simulink model "cantxrx"  (R2020b)
settings: Solver=FixedStepDiscrete  StartTime=0.0  StopTime=Inf  FixedStep=1e-3  RelTol=1e-3  EnableMultiTasking=on
model workspace (MAT data in the model file):
  state_control = Simulink.Signal
  state_control.DataType = 'uint8'
  state_control.Dimensions = -1
  state_control.DimensionsMode = 'Fixed'
  state_control.Complexity = 'real'
  state_control.SampleTime = -1
  state_control.SamplingMode = 'auto'
  state_control.InitialValue = '99'
libraries: simulink x12, hdlsllib x10, c280xlib x3, canmsglib x2, c2837xDlib x2, c2000lib x1
settings Model: ExtModeTrigDuration=8  OrderedModelArguments=off  Creator=sgcesuser2  LastModifiedBy=sgcesuser2
settings SolverCC: AutoInsertRateTranBlk=on
settings OptimizationCC: DefaultUnderspecifiedDataType=single  EnhancedBackFolding=on  PassReuseOutputArgsAs=Individual arguments  MaxStackSize=1024  OptimizeBlockOrder=speed  DifferentSizesBufferReuse=on  OptimizationCustomize=off  DenormalBehavior=FlushToZero  EfficientTunableParamExpr=on
settings DebuggingCC: ParameterTunabilityLossMsg=error
settings HardwareCC: ProdBitPerChar=16  ProdBitPerInt=16  ProdBitPerPointer=32  ProdBitPerSizeT=32  ProdBitPerPtrDiffT=32  ProdLargestAtomicInteger=Integer  ProdLargestAtomicFloat=None  ProdWordSize=16  ProdLongLongMode=on  ProdHWDeviceType=Texas Instruments->C2000
settings SFSimCC: MATLABDynamicMemAlloc=off
settings RTWCC: Description=Embedded Coder  SystemTargetFile=ert.tlc  HardwareBoard=TI Delfino F28379D LaunchPad  TemplateMakefile=ert_default_tmf  CustomHeaderCode="#include \"can_defines.h\""  Toolchain=Texas Instruments Code Composer Studio (C2000)
settings CodeAppCC: ForceParamTrailComments=on  IgnoreCustomStorageClasses=off  OperatorAnnotations=on  SimulinkDataObjDesc=on  SFDataObjDesc=on  InsertBlockDesc=on
settings ERTTargetCC: CodeReplacementLibrary=TI C28x  ExtModeTransport=3  ExtModeStaticAllocSize=10000

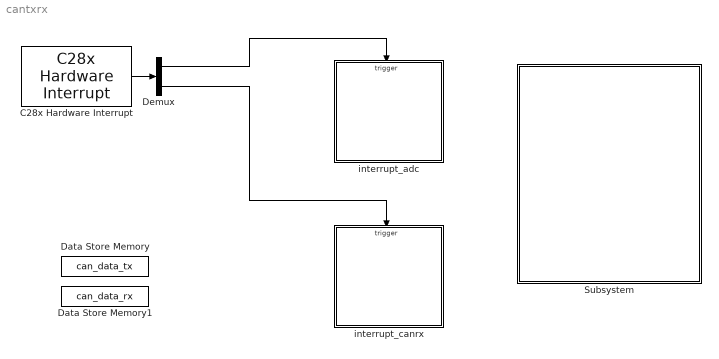
== system cantxrx ==
  C28x Hardware Interrupt : c2000lib/Scheduling/C28x Hardware Interrupt  irqnumbers=[1 9]  pienumbers=[1 7]  irqpriorities=[30 26]  irqpreempts=[0 1]  showinput=off  dspchiptype=C280X
      settings: SourceProductBaseCode=TIC2000
  Data Store Memory : DataStoreMemory  DataStoreName=can_data_tx  ReadBeforeWriteMsg=warning  WriteAfterWriteMsg=warning  WriteAfterReadMsg=warning  ShowAdditionalParam=off  Dimensions=[1 8]
  Data Store Memory1 : DataStoreMemory  DataStoreName=can_data_rx  ReadBeforeWriteMsg=warning  WriteAfterWriteMsg=warning  WriteAfterReadMsg=warning  ShowAdditionalParam=off  Dimensions=[1 8]
  Demux : Demux  Outputs=2
  Subsystem : Subsystem  TreatAsAtomicUnit=on  SystemSampleTime=1
  interrupt_adc : Subsystem  TreatAsAtomicUnit=on
      settings: RTWFcnNameOpts=Use subsystem name  RTWFileNameOpts=Use subsystem name
  interrupt_canrx : Subsystem  TreatAsAtomicUnit=on
      settings: RTWFcnNameOpts=Use subsystem name  RTWFileNameOpts=Use subsystem name
  wires:
  Demux/2 -> interrupt_canrx/Trigger
  Demux/1 -> interrupt_adc/Trigger
  C28x Hardware Interrupt/1 -> Demux/1

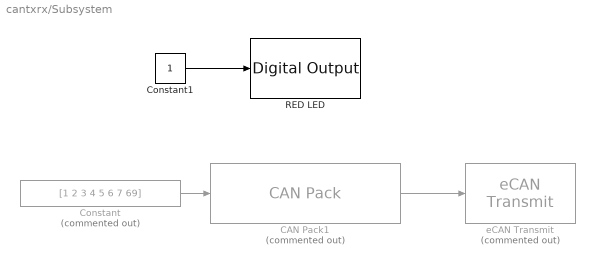
== system cantxrx/Subsystem ==
  CAN Pack1 : canmsglib/CAN Pack  Commented=on  MsgList=(none)  MsgName=CAN Msg  MsgIDType=Standard (11-bit identifier)  MsgIdentifier=2  MsgLength=8  Remote=off  ApplyMinMax=off  BusOutput=off  SignalInfo={}
      settings: SourceProductBaseCode=ME,XP,VN  DataFormat=raw data
  Constant : Constant  Commented=on  Value=[1 2 3 4 5 6 7 69]  OutDataTypeStr=uint8  SampleTime=-1
  Constant1 : Constant
  RED LED : c2837xDlib/Digital Output  GPIO_Number=GPIO32~GPIO39  GPIO_Bit0=off  GPIO_BIT0_Toggle=off  GPIO_Bit1=off  GPIO_BIT1_Toggle=off  GPIO_Bit2=on  GPIO_BIT2_Toggle=on  GPIO_Bit3=off  GPIO_BIT3_Toggle=off  GPIO_Bit4=off  GPIO_BIT4_Toggle=off  GPIO_Bit5=off  GPIO_BIT5_Toggle=off  GPIO_Bit6=off  GPIO_BIT6_Toggle=off  GPIO_Bit7=off  GPIO_BIT7_Toggle=off
      settings: SourceProductBaseCode=TIC2000
  eCAN Transmit : c280xlib/eCAN Transmit  Commented=on  chipFamily=C280x  useModule=eCAN_B  mailboxNo=1  messageID=bin2dec('111000111')  messageType=Standard (11-bit identifier)  enableBlockingMode=off  postInterrupt=off  interruptLine=0
      settings: SourceProductBaseCode=TIC2000
  wires:
  CAN Pack1/1 -> eCAN Transmit/1
  Constant/1 -> CAN Pack1/1
  Constant1/1 -> RED LED/1

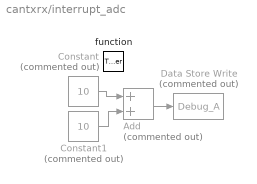
== system cantxrx/interrupt_adc ==
  function : TriggerPort  TriggerType=function-call  VariantControl=Variant
  Add : Sum  Commented=on
  Constant : Constant  Commented=on  Value=10  OutDataTypeStr=uint16
  Constant1 : Constant  Commented=on  Value=10  OutDataTypeStr=uint16
  Data Store Write : DataStoreWrite  Commented=on  DataStoreName=Debug_A
  wires:
  Constant/1 -> Add/1
  Constant1/1 -> Add/2
  Add/1 -> Data Store Write/1

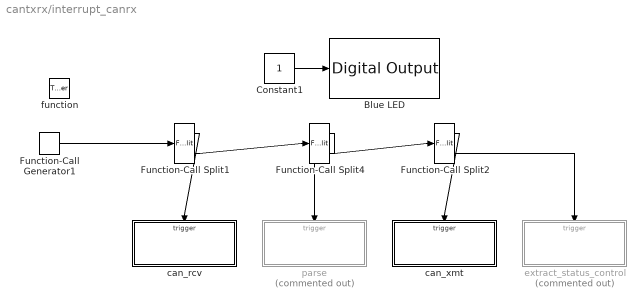
== system cantxrx/interrupt_canrx ==
  function : TriggerPort  TriggerType=function-call  VariantControl=Variant
  Blue LED : c2837xDlib/Digital Output  GPIO_Number=GPIO24~GPIO31  GPIO_Bit0=off  GPIO_BIT0_Toggle=off  GPIO_Bit1=off  GPIO_BIT1_Toggle=off  GPIO_Bit2=off  GPIO_BIT2_Toggle=off  GPIO_Bit3=off  GPIO_BIT3_Toggle=off  GPIO_Bit4=off  GPIO_BIT4_Toggle=off  GPIO_Bit5=off  GPIO_BIT5_Toggle=off  GPIO_Bit6=off  GPIO_BIT6_Toggle=off  GPIO_Bit7=on  GPIO_BIT7_Toggle=on
      settings: SourceProductBaseCode=TIC2000
  Constant1 : Constant
  Function-Call Generator1 : simulink/Ports & Subsystems/Function-Call Generator  sample_time=-1  numberOfIterations=1  DisallowWideOutput=off
  Function-Call Split1 : FunctionCallSplit  NumOutputPorts=2
  Function-Call Split2 : FunctionCallSplit  NumOutputPorts=2
  Function-Call Split4 : FunctionCallSplit  NumOutputPorts=2
  can_rcv : Subsystem  TreatAsAtomicUnit=on
  can_xmt : Subsystem  TreatAsAtomicUnit=on
  extract_status_control : Subsystem  Commented=on  TreatAsAtomicUnit=on
  parse : Subsystem  Commented=on  TreatAsAtomicUnit=on
  wires:
  Function-Call Split4/2 -> Function-Call Split2/1
  Function-Call Split2/2 -> extract_status_control/Trigger
  Function-Call Generator1/1 -> Function-Call Split1/1
  Function-Call Split2/1 -> can_xmt/Trigger
  Function-Call Split1/2 -> Function-Call Split4/1
  Function-Call Split1/1 -> can_rcv/Trigger
  Function-Call Split4/1 -> parse/Trigger
  Constant1/1 -> Blue LED/1

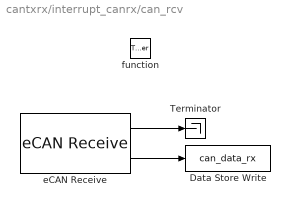
== system cantxrx/interrupt_canrx/can_rcv ==
  function : TriggerPort  TriggerType=function-call  VariantControl=Variant
  Data Store Write : DataStoreWrite  DataStoreName=can_data_rx  DataStoreElements=can_data_rx
  Terminator : Terminator
  eCAN Receive : c280xlib/eCAN Receive  chipFamily=C280x  useModule=eCAN_B  mailboxNo=0  messageID=bin2dec('000000001')  messageType=Standard (11-bit identifier)  sampleTime=-1  dataType=uint8  initValue=0  outputMessageLength=off  outputMessageTimeStamp=off  postInterrupt=on  interruptLine=0
      settings: SourceProductBaseCode=TIC2000
  wires:
  eCAN Receive/1 -> Terminator/1
  eCAN Receive/2 -> Data Store Write/1

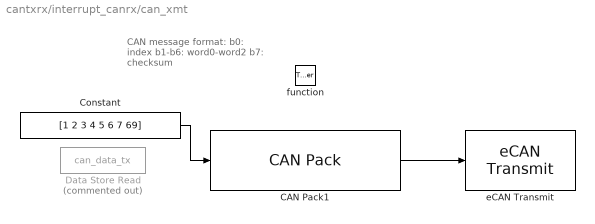
== system cantxrx/interrupt_canrx/can_xmt ==
  note: CAN message format:
      | b0: index
      | b1-b6: word0-word2
      | b7: checksum
  function : TriggerPort  TriggerType=function-call  VariantControl=Variant
  CAN Pack1 : canmsglib/CAN Pack  MsgList=(none)  MsgName=CAN Msg  MsgIDType=Standard (11-bit identifier)  MsgIdentifier=2  MsgLength=8  Remote=off  ApplyMinMax=off  BusOutput=off  SignalInfo={}
      settings: SourceProductBaseCode=ME,XP,VN  DataFormat=raw data
  Constant : Constant  Value=[1 2 3 4 5 6 7 69]  OutDataTypeStr=uint8  SampleTime=-1
  Data Store Read : DataStoreRead  Commented=on  DataStoreName=can_data_tx
  eCAN Transmit : c280xlib/eCAN Transmit  chipFamily=C280x  useModule=eCAN_B  mailboxNo=1  messageID=bin2dec('111000111')  messageType=Standard (11-bit identifier)  enableBlockingMode=off  postInterrupt=off  interruptLine=0
      settings: SourceProductBaseCode=TIC2000
  wires:
  CAN Pack1/1 -> eCAN Transmit/1
  Constant/1 -> CAN Pack1/1

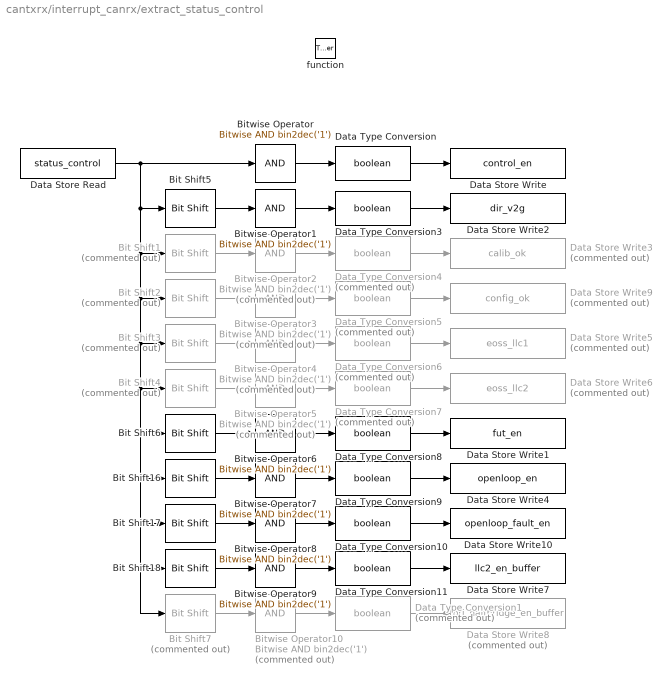
== system cantxrx/interrupt_canrx/extract_status_control ==
  function : TriggerPort  TriggerType=function-call  VariantControl=Variant
  Bit Shift1 : hdlsllib/Logic and Bit Operations/Bit Shift  Commented=on  mode=Shift Right Logical  N=2
  Bit Shift16 : hdlsllib/Logic and Bit Operations/Bit Shift  mode=Shift Right Logical  N=7
  Bit Shift17 : hdlsllib/Logic and Bit Operations/Bit Shift  mode=Shift Right Logical  N=8
  Bit Shift18 : hdlsllib/Logic and Bit Operations/Bit Shift  mode=Shift Right Logical  N=9
  Bit Shift2 : hdlsllib/Logic and Bit Operations/Bit Shift  Commented=on  mode=Shift Right Logical  N=3
  Bit Shift3 : hdlsllib/Logic and Bit Operations/Bit Shift  Commented=on  mode=Shift Right Logical  N=4
  Bit Shift4 : hdlsllib/Logic and Bit Operations/Bit Shift  Commented=on  mode=Shift Right Logical  N=5
  Bit Shift5 : hdlsllib/Logic and Bit Operations/Bit Shift  mode=Shift Right Logical  N=1
  Bit Shift6 : hdlsllib/Logic and Bit Operations/Bit Shift  mode=Shift Right Logical  N=6
  Bit Shift7 : hdlsllib/Logic and Bit Operations/Bit Shift  Commented=on  mode=Shift Right Logical  N=10
  Bitwise Operator{,1,6..9} (6 alike) : simulink/Logic and Bit Operations/Bitwise Operator  logicop=AND  UseBitMask=on  BitMask=bin2dec('1')  BitMaskRealWorld=Stored Integer
  Bitwise Operator{2..5,10} (5 alike) : simulink/Logic and Bit Operations/Bitwise Operator  Commented=on  logicop=AND  UseBitMask=on  BitMask=bin2dec('1')  BitMaskRealWorld=Stored Integer
  Data Store Read : DataStoreRead  DataStoreName=status_control
  Data Store Write : DataStoreWrite  DataStoreName=control_en
  Data Store Write1 : DataStoreWrite  DataStoreName=fut_en
  Data Store Write10 : DataStoreWrite  DataStoreName=openloop_fault_en
  Data Store Write2 : DataStoreWrite  DataStoreName=dir_v2g
  Data Store Write3 : DataStoreWrite  Commented=on  DataStoreName=calib_ok
  Data Store Write4 : DataStoreWrite  DataStoreName=openloop_en
  Data Store Write5 : DataStoreWrite  Commented=on  DataStoreName=eoss_llc1
  Data Store Write6 : DataStoreWrite  Commented=on  DataStoreName=eoss_llc2
  Data Store Write7 : DataStoreWrite  DataStoreName=llc2_en_buffer
  Data Store Write8 : DataStoreWrite  Commented=on  DataStoreName=pri_halfbridge_en_buffer
  Data Store Write9 : DataStoreWrite  Commented=on  DataStoreName=config_ok
  Data Type Conversion{,3,8..11} (6 alike) : DataTypeConversion  OutDataTypeStr=boolean
  Data Type Conversion{1,4..7} (5 alike) : DataTypeConversion  Commented=on  OutDataTypeStr=boolean
  wires:
  Bitwise Operator/1 -> Data Type Conversion/1
  Bit Shift5/1 -> Bitwise Operator1/1
  Bit Shift1/1 -> Bitwise Operator2/1
  Bit Shift2/1 -> Bitwise Operator3/1
  Bit Shift3/1 -> Bitwise Operator4/1
  Bit Shift4/1 -> Bitwise Operator5/1
  Bit Shift6/1 -> Bitwise Operator6/1
  Bit Shift16/1 -> Bitwise Operator7/1
  Bit Shift17/1 -> Bitwise Operator8/1
  Bit Shift18/1 -> Bitwise Operator9/1
  Bitwise Operator1/1 -> Data Type Conversion3/1
  Bitwise Operator2/1 -> Data Type Conversion4/1
  Bitwise Operator3/1 -> Data Type Conversion5/1
  Data Type Conversion3/1 -> Data Store Write2/1
  Data Type Conversion4/1 -> Data Store Write3/1
  Bitwise Operator4/1 -> Data Type Conversion6/1
  Bitwise Operator5/1 -> Data Type Conversion7/1
  Bitwise Operator6/1 -> Data Type Conversion8/1
  Bitwise Operator7/1 -> Data Type Conversion9/1
  Bitwise Operator8/1 -> Data Type Conversion10/1
  Bitwise Operator9/1 -> Data Type Conversion11/1
  Bitwise Operator10/1 -> Data Type Conversion1/1
  Data Store Read/1 -> Bit Shift17/1, Bit Shift7/1, Bit Shift18/1, Bit Shift16/1, Bit Shift6/1, Bit Shift4/1, Bit Shift3/1, Bit Shift2/1, Bit Shift1/1, Bit Shift5/1, Bitwise Operator/1
  Bit Shift7/1 -> Bitwise Operator10/1
  Data Type Conversion/1 -> Data Store Write/1
  Data Type Conversion5/1 -> Data Store Write9/1
  Data Type Conversion6/1 -> Data Store Write5/1
  Data Type Conversion7/1 -> Data Store Write6/1
  Data Type Conversion8/1 -> Data Store Write1/1
  Data Type Conversion9/1 -> Data Store Write4/1
  Data Type Conversion10/1 -> Data Store Write10/1
  Data Type Conversion11/1 -> Data Store Write7/1
  Data Type Conversion1/1 -> Data Store Write8/1

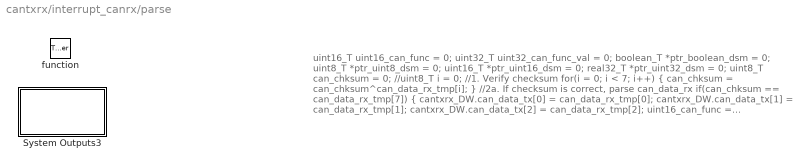
== system cantxrx/interrupt_canrx/parse ==
  note: uint16_T uint16_can_func = 0;
      | uint32_T uint32_can_func_val = 0;
      | boolean_T *ptr_boolean_dsm = 0;
      | uint8_T *ptr_uint8_dsm = 0;
      | uint16_T *ptr_uint16_dsm = 0;
      | real32_T *ptr_uint32_dsm = 0;
      | uint8_T can_chksum = 0;
      | //uint8_T i = 0;
      | //1. Verify checksum
      | for(i = 0; i < 7; i++)
      | {
      | 	can_chksum = can_chksum^can_data_rx_tmp[i];
      | }
      | //2a. If checksum is correct, parse can_data_rx
      | if(can_chksum == can_data_rx_tmp[7])
      | {
      | 	cantxrx_DW.can_data_tx[0] = can_data_rx_tmp[0];
      | 	cantxrx_DW.can_data_tx[1] = can_data_rx_tmp[1];
      | 	cantxrx_DW.can_data_tx[2] = can_data_rx_tmp[2];
      | 	uint16_can_func = (can_data_rx_tmp[2]<<8) | can_data_rx_tmp[1];
      | 	uint32_can_func_val = (can_data_rx_tmp[6]<<24) | (can_data_rx_tmp[5]<<16) | (can_data_rx_tmp[4]<<8) | can_data_rx_tmp[3];
      | 	if(uint16_can_func == 0x000)
      |          {
      | 	   ptr_uint8_dsm = &dsm_0000;
      |           sendUint8CanDataTx();
      |          }
      | 	else
      |          {sendErrorFunc(); }
      | }
      | //2b. If checksum error
      | else
      | {
      | 	sendErrorChksum();
      | }
      | //3. Caclulate checksum for can_data_tx
      | cantxrx_DW.can_data_tx[7] = 0;
      | for(i = 0; i < 7; i++){
      | 	cantxrx_DW.can_data_tx[7] = cantxrx_DW.can_data_tx[7]^cantxrx_DW.can_data_tx[i];
      | }
  function : TriggerPort  TriggerType=function-call  VariantControl=Variant
  System Outputs3 : Subsystem  mask(System Outputs){ShowInLibBrowser=0}
      mask prompts: ShowInLibBrowser "Simulink:masks:CustCodeMaskParam1_MP"
      settings: CopyFcn=cccopyfcn(gcb)  OpenFcn=ccopenfcn('System Outputs Function')
      mask Help: eval('feval(''rtwprivate'',''rtwhelpview'',''rtw_sys_outputs_block'')');
      mask Display: disp('System\nOutputs');

== system cantxrx/interrupt_canrx/parse/System Outputs3 ==
